simulink model "Torque_Control_22"  (R2023b)
settings: Solver=FixedStepAuto  StartTime=0.0  StopTime=10.0  RelTol=1e-3
libraries: simulink x15, peGeneralControl x6
(part 1 of 6)
settings Model: Creator=cspt  LastModifiedBy=Mátyás
settings SolverCC: AlgebraicLoopSolver=TrustRegion
settings DataIOCC: ReturnWorkspaceOutputs=off
settings DebuggingCC: UnconnectedInputMsg=warning  UnconnectedOutputMsg=warning  UnconnectedLineMsg=warning  ArithmeticOperatorsInVariantConditions=warning
settings ModelReferenceCC: EnableRefExpFcnMdlSchedulingChecks=on
settings SFSimCC: SimUseLocalCustomCode=off  CustomCodeUndefinedFunction=UseInterfaceOnly
settings RTWCC: Description=INTECRIO Real-Time Target  SystemTargetFile=irt.tlc  TemplateMakefile=irt_default_tmf  RTWUseLocalCustomCode=off
settings STFCustomTargetCC: UtilityFuncGeneration=Shared location  GRTInterface=on  SystemTargetFile=irt.tlc
settings GRTTargetCC: UtilityFuncGeneration=Shared location  ParMdlRefBuildCompliant=off  CompOptLevelCompliant=off  ConcurrentExecutionCompliant=off  CombineOutputUpdateFcns=off  MatFileLogging=off  CPPClassGenCompliant=off  GRTInterface=on  UseToolchainInfoCompliant=off  GenerateASAP2=on

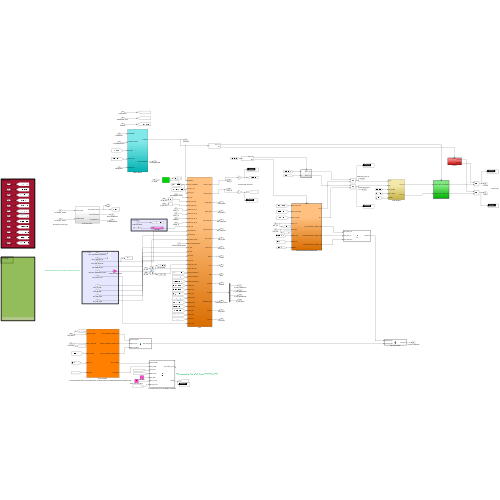
[thumbnail: Simulink's stored preview of the top-level diagram]
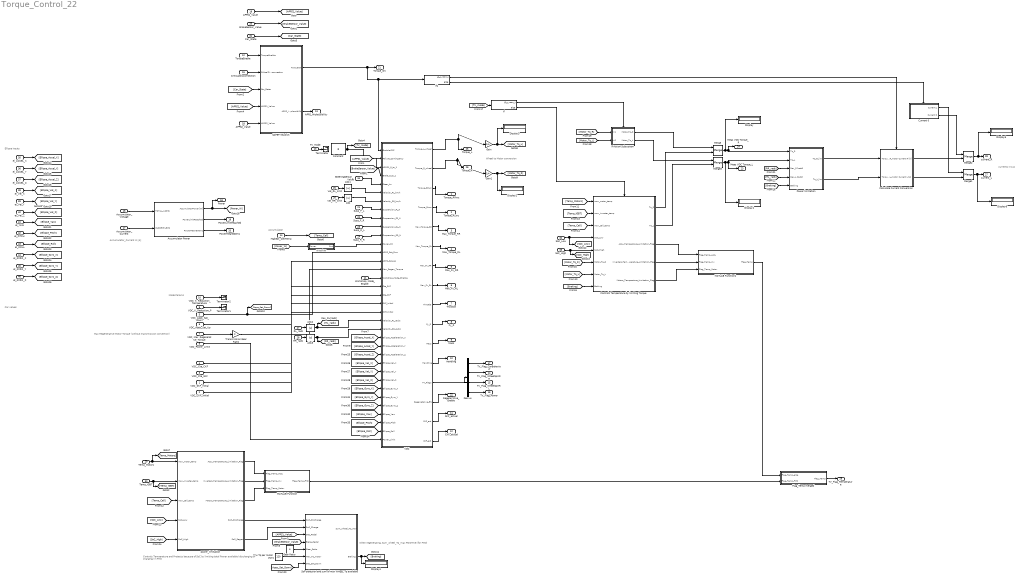
== system Torque_Control_22 ==
  note: Ellipse Inputs
  note: Accumulator_Current in [A]
  note: When regenerating, Sum_wheel_Tq_max POSITIVE (for FM0)
  note: Wheel to Motor conversion
  note: Max Regenerative Motor Torque (without transmission convertion)
  note: Controls Temperature and Protects because of SoC by limiting total Power available (discharging or charging) in FM0
  note: Mode Params
  note: Accumulator
  note: currents in [A]
  note: Car values
  VDC_SKF_Initial : Inport
  VDC_CKF_Initial : Inport  Port=2
  VDC_Cte_SKF : Inport  Port=3
  VDC_Cte_CKF : Inport  Port=4
  VDC_Apps_Sat_Down : Inport  Port=5
  VDC_Apps_Sat_Up : Inport  Port=6
  VDC_Max_Regenerative_Torque : Inport  Port=7
  VDC_Power_Limit : Inport  Port=8
  VDC_K_Reduction_P : Inport  Port=9
  VDC_K_Reduction_Temperature : Inport  Port=10
  Workshop_Mode_Enable : Inport  Port=11
  TorqueEnable : Inport  Port=12
  TV_Mode : Inport  Port=13
  Highest_CellTemp : Inport  Port=14
  CriticalDisconnection : Inport  Port=15
  Accumulator_Voltage : Inport  Port=16
  Accumulator_Current : Inport  Port=17
  APPS2_Value : Inport  Port=18
  APPS1_Value : Inport  Port=19
  BrakeSensor_Value : Inport  Port=20
  Susp_F_L : Inport  Port=21
  Susp_F_R : Inport  Port=22
  Susp_R_L : Inport  Port=23
  Susp_R_R : Inport  Port=24
  Vel_RL_kmh : Inport  Port=25
  Vel_RR_kmh : Inport  Port=26
  RL_rads : Inport  Port=27
  RR_rads : Inport  Port=28
  Temp_Motors : Inport  Port=29
  Temp_IGBT : Inport  Port=30
  Car_State : Inport  Port=31
  SoC_Low : Inport  Port=32
  SoC_High : Inport  Port=33
  SteeringSensor_Value : Inport  Port=34
  el_ACCEL_X : Inport  Port=35
  el_ACCEL_Y : Inport  Port=36
  el_ACCEL_Z : Inport  Port=37
  el_Vel_X : Inport  Port=38
  el_Vel_Y : Inport  Port=39
  el_Vel_Z : Inport  Port=40
  el_YAW : Inport  Port=41
  el_PITCH : Inport  Port=42
  el_ROLL : Inport  Port=43
  el_GYRO_X : Inport  Port=44
  el_GYRO_Y : Inport  Port=45
  el_GYRO_Z : Inport  Port=46
  Abs{,1..3} (4 alike) : Abs  SaturateOnIntegerOverflow=off
  Accumulator Power : Subsystem
  Calculate Current Conversion : Subsystem
  Constant : Constant  Value=3
  Controls Temperature by limiting Torque : Subsystem  TreatAsAtomicUnit=on
  Current 0 : Subsystem  TreatAsAtomicUnit=on
  Demux : Demux
  Display{,1..6} (7 alike) : Display
  Flag_Temp merged : MATLAB Function  TreatAsAtomicUnit=on
  Gain : Gain  Gain=1/4
  Gain1 : Gain  Gain=1/4
  Gear Ratio : Constant  Value=4
  If : If  IfExpression=u1 == 1
  If Action Subsystem : Subsystem  TreatAsAtomicUnit=on
  If1 : If  IfExpression=u1 == 1
  MATLAB Function : MATLAB Function  TreatAsAtomicUnit=on
  MATLAB Function1 : MATLAB Function  TreatAsAtomicUnit=on
  Max Tq per motor [Nm] : Constant  Value=120
  Merge{,1..3} (4 alike) : Merge
  Power limitation : Subsystem
  SAFETY BLOCK : Subsystem
  SoP selection and sum of max WHEEL Tq available : MATLAB Function  TreatAsAtomicUnit=on
  Terminator : Terminator
  Terminator1 : Terminator
  Terminator2 : Terminator
  Transmission Gear Ratio : Gain  Gain=4
  VDC : Subsystem
  W to kW : Subsystem
  power_limitation : Subsystem
  Torque_RRwc : Outport  VectorParamsAs1DForOutWhenUnconnected=off
  Torque_RLwc : Outport  Port=2  VectorParamsAs1DForOutWhenUnconnected=off
  Max_Torque_RR : Outport  Port=3  VectorParamsAs1DForOutWhenUnconnected=off
  Max_Torque_RL : Outport  Port=4  VectorParamsAs1DForOutWhenUnconnected=off
  Max_Fx_RR : Outport  Port=5  VectorParamsAs1DForOutWhenUnconnected=off
  Max_Fx_RL : Outport  Port=6  VectorParamsAs1DForOutWhenUnconnected=off
  Throttle : Outport  Port=7  VectorParamsAs1DForOutWhenUnconnected=off
  Fy_R : Outport  Port=8  VectorParamsAs1DForOutWhenUnconnected=off
  Mass : Outport  Port=9  VectorParamsAs1DForOutWhenUnconnected=off
  Handling : Outport  Port=10  VectorParamsAs1DForOutWhenUnconnected=off
  SKF_actual : Outport  Port=11  VectorParamsAs1DForOutWhenUnconnected=off
  CKF_actual : Outport  Port=12  VectorParamsAs1DForOutWhenUnconnected=off
  APPS_Implausibility : Outport  Port=13  VectorParamsAs1DForOutWhenUnconnected=off
  TV_Flag_WheelSpinRR : Outport  Port=14  VectorParamsAs1DForOutWhenUnconnected=off
  TV_Flag_WheelSpinRL : Outport  Port=15  VectorParamsAs1DForOutWhenUnconnected=off
  TV_Flag_Power : Outport  Port=16  VectorParamsAs1DForOutWhenUnconnected=off
  TV_Flag_CarBehaviour : Outport  Port=17  VectorParamsAs1DForOutWhenUnconnected=off
  Power : Outport  Port=18  VectorParamsAs1DForOutWhenUnconnected=off
  PowerLimitReached : Outport  Port=19  VectorParamsAs1DForOutWhenUnconnected=off
  PowerMean500ms : Outport  Port=20  VectorParamsAs1DForOutWhenUnconnected=off
  Torque_OK : Outport  Port=21  VectorParamsAs1DForOutWhenUnconnected=off
  Regenerative_Enable : Outport  Port=22  VectorParamsAs1DForOutWhenUnconnected=off
  Meas VDC Torque_L : Outport  Port=23  VectorParamsAs1DForOutWhenUnconnected=off
  Meas VDC Torque_R : Outport  Port=24  VectorParamsAs1DForOutWhenUnconnected=off
  Torque_L : Outport  Port=25  VectorParamsAs1DForOutWhenUnconnected=off
  Torque_R : Outport  Port=26  VectorParamsAs1DForOutWhenUnconnected=off
  current_L : Outport  Port=27  VectorParamsAs1DForOutWhenUnconnected=off
  current_R : Outport  Port=28  VectorParamsAs1DForOutWhenUnconnected=off
  TV_Flag_Temperature : Outport  Port=29  VectorParamsAs1DForOutWhenUnconnected=off
  wires:
  Accumulator Power/1(AccumulatorPower [W]) -> [Power_W], Power/1
  Workshop_Mode_Enable/1 -> VDC/16(Workshop_Mode_Enable)
  SAFETY BLOCK/2(APPS_Implausibility) -> APPS_Implausibility/1
  VDC_Cte_SKF/1 -> VDC/18(Cte_CKF)
  VDC_Apps_Sat_Down/1 -> VDC/13(APPS_Sat_Dwn), [Apps_Sat_Down]
  VDC_Cte_CKF/1 -> VDC/17(Cte_SKF)
  VDC_SKF_Initial/1 -> VDC/19(SKF_Initial)
  VDC/3(Torque_RRwc) -> Torque_RRwc/1
  Highest_CellTemp/1 -> [Temp_Cell]
  [Car_State] -> SAFETY BLOCK/3(Car_State)
  Accumulator_Current/1 -> Accumulator Power/2(CURRENT_BMS)
  Accumulator Power/3(PowerMean500ms) -> PowerMean500ms/1
  Demux/1 -> TV_Flag_CarBehaviour/1
  VDC/14(Regenetarive_EN) -> Regenerative_Enable/1
  VDC/10(Fy_R) -> Fy_R/1
  If1/2 -> Current 0/Action
  If1/1 -> Calculate Current Conversion/Action
  VDC_Apps_Sat_Up/1 -> VDC/14(APPS_Sat_Up)
  TorqueEnable/1 -> SAFETY BLOCK/1(TorqueEnable)
  VDC/5(Max_Torque_RR) -> Max_Torque_RR/1
  Accumulator_Voltage/1 -> Accumulator Power/1(TOTAL_V_BMS)
  Accumulator Power/2(PowerLimitReached) -> PowerLimitReached/1
  VDC/7(Max_Fx_RR) -> Max_Fx_RR/1
  VDC/8(Max_Fx_RL) -> Max_Fx_RL/1
  VDC_CKF_Initial/1 -> VDC/20(CKF_Initial)
  Demux/2 -> TV_Flag_WheelSpinRR/1
  VDC/9(Throttle) -> Throttle/1
  Demux/3 -> TV_Flag_WheelSpinRL/1
  [Power_W] -> W to kW/1(Power)
  CriticalDisconnection/1 -> SAFETY BLOCK/2(CriticalDisconnection)
  VDC/11(Mass) -> Mass/1
  VDC/16(CKF_act) -> CKF_actual/1
  VDC/12(Handling) -> Handling/1
  VDC/13(TV_Flags) -> Demux/1
  VDC/6(Max_Torque_RL) -> Max_Torque_RL/1
  VDC/15(SKF_act) -> SKF_actual/1
  VDC/4(Torque_RLwc) -> Torque_RLwc/1
  APPS1_Value/1 -> [APPS1_Value]
  BrakeSensor_Value/1 -> [BrakeSensor_Value]
  Susp_F_L/1 -> VDC/8(Suspension_FL_N)
  Susp_F_R/1 -> VDC/9(Suspension_FR_N)
  Susp_R_L/1 -> VDC/10(Suspension_RL_N)
  Susp_R_R/1 -> VDC/11(Suspension_RR_N)
  APPS2_Value/1 -> SAFETY BLOCK/5(APPS2_Value)
  Car_State/1 -> [Car_State]
  Abs/1 -> VDC/7(Velocity_RR_km/h)
  Abs1/1 -> VDC/6(Velocity_RL_km/h)
  Abs2/1 -> [RL_rads], VDC/21(Velocity_RL_rad/s)
  Merge1/1 -> Display6/1, current_L/1
  Merge2/1 -> Display5/1, current_R/1
  W to kW/1(Out) -> VDC/12(Power_kW)
  VDC/2(Torque_R_wheel) -> Torque_R/1, Gain1/1
  VDC_K_Reduction_P/1 -> Terminator1/1
  VDC_K_Reduction_Temperature/1 -> Terminator2/1
  Demux/4 -> TV_Flag_Power/1
  MATLAB Function/1(Flag_Temp_FM0) -> Flag_Temp merged/2(Flag_Temp_FM0)
  Abs3/1 -> [RR_rads], VDC/22(Velocity_RR_rad/s)
  Current 0/1(Current L) -> Merge1/1
  Calculate Current Conversion/2(Current L [A]) -> Merge1/2
  Transmission Gear Ratio/1 -> VDC/15(Max_Regen_Torque)
  Temp_Motors/1 -> power_limitation/1(max_motor_temp), [Temp_Motors]
  Temp_IGBT/1 -> power_limitation/2(max_inverter_temp), [Temp_IGBT]
  [Temp_Cell] -> power_limitation/3(max_cell_temp)
  [SoC_Low] -> power_limitation/4(SoC_Low)
  [SoC_High] -> power_limitation/5(SoC_High)
  power_limitation/2(Inverters_Temperature_Limitation_Flag) -> MATLAB Function/2(Flag_Temp_Inv)
  power_limitation/1(Accu_Temperature_Limitation_Flag) -> MATLAB Function/1(Flag_Temp_Accu)
  power_limitation/3(Motors_Temperature_Limitation_Flag) -> MATLAB Function/3(Flag_Temp_Motor)
  VDC/1(Torque_L_wheel) -> Gain/1, Torque_L/1
  power_limitation/4(SoP_Discharge) -> SoP selection and sum of max WHEEL Tq available/1(SoP_Discharge)
  power_limitation/5(SoP_Regen) -> SoP selection and sum of max WHEEL Tq available/2(SoP_Charge)
  [APPS1_Value] -> VDC/3(APPS1_0_to_1)
  [BrakeSensor_Value] -> VDC/4(Brake_0_to_1)
  [APPS1_Value] -> SoP selection and sum of max WHEEL Tq available/3(Gas_Pedal)
  [BrakeSensor_Value] -> SoP selection and sum of max WHEEL Tq available/4(Brake_Pedal)
  Gear Ratio/1 -> SoP selection and sum of max WHEEL Tq available/5(Gear_Ratio)
  Max Tq per motor [Nm]/1 -> SoP selection and sum of max WHEEL Tq available/6(Max_Tq_motor)
  [Motor_Tq_R] -> Controls Temperature by limiting Torque/6(Motor_Tq_R)
  [Motor_Tq_L] -> Controls Temperature by limiting Torque/7(Motor_Tq_L)
  MATLAB Function1/1(Flag_Temp) -> Flag_Temp merged/1(Flag_Temp_else)
  [Temp_Motors] -> Controls Temperature by limiting Torque/1(max_motor_temp)
  SoC_High/1 -> [SoC_High], Controls Temperature by limiting Torque/5(SoC_High)
  [Temp_Cell] -> Controls Temperature by limiting Torque/3(max_cell_temp)
  Controls Temperature by limiting Torque/4(Inverters_Temperature_Limitation_Flag) -> MATLAB Function1/2(Flag_Temp_Inv)
  Controls Temperature by limiting Torque/3(Accu_Temperature_Limitation_Flag) -> MATLAB Function1/1(Flag_Temp_Accu)
  [TV_mode] -> If/1
  Gain1/1 -> Display2/1, [Motor_Tq_R]
  Gain/1 -> Display3/1, [Motor_Tq_L]
  Merge3/1 -> Display1/1, Power limitation/2(Tq_L), Meas VDC Torque_L/1
  If/1 -> If Action Subsystem/Action
  [Motor_Tq_R] -> If Action Subsystem/1(In1)
  [Motor_Tq_L] -> If Action Subsystem/2(In2)
  Merge/1 -> Display/1, Power limitation/1(Tq_R), Meas VDC Torque_R/1
  If/2 -> Controls Temperature by limiting Torque/Action
  If Action Subsystem/1(Motor_Tq_R) -> Merge/1
  If Action Subsystem/2(Motor_Tq_L) -> Merge3/1
  Controls Temperature by limiting Torque/1(Tq_R) -> Merge/2
  Controls Temperature by limiting Torque/2(Tq_L) -> Merge3/2
  Flag_Temp merged/1(Flag_Temp) -> TV_Flag_Temperature/1
  Vel_RL_kmh/1 -> Abs1/1
  Vel_RR_kmh/1 -> Abs/1
  RL_rads/1 -> Abs2/1
  RR_rads/1 -> Abs3/1
  VDC_Max_Regenerative_Torque/1 -> Transmission Gear Ratio/1
  SoC_Low/1 -> [SoC_Low], Controls Temperature by limiting Torque/4(SoC_Low)
  [Temp_IGBT] -> Controls Temperature by limiting Torque/2(max_inverter_temp)
  Controls Temperature by limiting Torque/5(Motors_Temperature_Limitation_Flag) -> MATLAB Function1/3(Flag_Temp_Motor)
  [Apps_Sat_Down] -> SoP selection and sum of max WHEEL Tq available/7(Gas_Sat_Down)
  SoP selection and sum of max WHEEL Tq available/2(Braking) -> Display4/1, [Braking]
  [Braking] -> Controls Temperature by limiting Torque/8(Braking)
  Calculate Current Conversion/1(Current R [A]) -> Merge2/2
  Current 0/2(Current R) -> Merge2/1
  SAFETY BLOCK/1(TorqueOK) -> If1/1, VDC/1(EnableVDC), Torque_OK/1
  [RR_rads] -> Power limitation/3(Rev_R [rads])
  [RL_rads] -> Power limitation/4(Rev_L [rads])
  [Braking] -> Power limitation/5(Braking)
  Power limitation/1(Tq_R_lim) -> Calculate Current Conversion/1(Torque_R_motor)
  Power limitation/2(Tq_L_lim) -> Calculate Current Conversion/2(Torque_L_motor)
  TV_Mode/1 -> Terminator/1
  Constant/1 -> [TV_mode], VDC/2(Failure_Contingency)
  SteeringSensor_Value/1 -> VDC/5(Steer_An)
  [APPS1_Value] -> SAFETY BLOCK/4(APPS1_Value)
  el_ACCEL_X/1 -> [Ellipse_Accel_X]
  el_ACCEL_Y/1 -> [Ellipse_Accel_Y]
  el_ACCEL_Z/1 -> [Ellipse_Accel_Z]
  el_Vel_Y/1 -> [Ellipse_Vel_Y]
  el_Vel_Z/1 -> [Ellipse_Vel_Z]
  el_Vel_X/1 -> [Ellipse_Vel_X]
  el_PITCH/1 -> [Ellipse_Pitch]
  el_ROLL/1 -> [Ellipse_Roll]
  el_GYRO_X/1 -> [Ellipse_Gyro_X]
  el_GYRO_Y/1 -> [Ellipse_Gyro_Y]
  el_GYRO_Z/1 -> [Ellipse_Gyro_Z]
  el_YAW/1 -> [Ellipse_Yaw]
  [Ellipse_Accel_X] -> VDC/23(Ellipse_Acceleration_X)
  [Ellipse_Accel_Y] -> VDC/24(Ellipse_Acceleration_Y)
  [Ellipse_Accel_Z] -> VDC/25(Ellipse_Acceleration_Z)
  [Ellipse_Vel_X] -> VDC/26(Ellipse_Vel_X)
  [Ellipse_Vel_Y] -> VDC/27(Ellipse_Vel_Y)
  [Ellipse_Vel_Z] -> VDC/28(Ellipse_Vel_Z)
  [Ellipse_Gyro_X] -> VDC/29(Ellipse_Gyro_X)
  [Ellipse_Gyro_Y] -> VDC/30(Ellipse_Gyro_Y)
  [Ellipse_Gyro_Z] -> VDC/31(Ellipse_Gyro_Z)
  [Ellipse_Yaw] -> VDC/32(Ellipse_Yaw)
  [Ellipse_Pitch] -> VDC/33(Ellipse_Pitch)
  [Ellipse_Roll] -> VDC/34(Ellipse_Roll)
  VDC_Power_Limit/1 -> VDC/35(Power_Limit)

== system Torque_Control_22/Accumulator Power ==
  TOTAL_V_BMS : Inport
  CURRENT_BMS : Inport  Port=2
  PowerLimitDetection : Subsystem  TreatAsAtomicUnit=on
  Product : Product
  AccumulatorPower [W] : Outport  VectorParamsAs1DForOutWhenUnconnected=off
  PowerLimitReached : Outport  Port=2  VectorParamsAs1DForOutWhenUnconnected=off
  PowerMean500ms : Outport  Port=3  VectorParamsAs1DForOutWhenUnconnected=off
  wires:
  Product/1 -> AccumulatorPower [W]/1, PowerLimitDetection/1(Power)
  PowerLimitDetection/1(PowerLimitReached) -> PowerLimitReached/1
  PowerLimitDetection/2(PowerMean500ms) -> PowerMean500ms/1
  TOTAL_V_BMS/1 -> Product/1
  CURRENT_BMS/1 -> Product/2

== system Torque_Control_22/Calculate Current Conversion ==
  Torque_R_motor : Inport
  Torque_L_motor : Inport  Port=2
  Action Port : ActionPort  ActionPortLabel=if { }
  Gain : Gain  Gain=-1
  KT_L_TORKY : Subsystem  TreatAsAtomicUnit=on
  KT_R_EMY : Subsystem  TreatAsAtomicUnit=on
  Current R [A] : Outport  VectorParamsAs1DForOutWhenUnconnected=off
  Current L [A] : Outport  Port=2  VectorParamsAs1DForOutWhenUnconnected=off
  wires:
  Torque_R_motor/1 -> KT_R_EMY/1(Torque)
  Torque_L_motor/1 -> KT_L_TORKY/1(Torque)
  Gain/1 -> Current L [A]/1
  KT_R_EMY/1(Current) -> Current R [A]/1
  KT_L_TORKY/1(Current) -> Gain/1

== system Torque_Control_22/Controls Temperature by limiting Torque ==
  note: Outputs:
      | Flags: 1 means power is being limited by temperature, 0 means not limited
      | SoP_discharge: State of Power for discharging
      | SoP_charge: State of Power for charging
  note: Inputs:
      | max_cell_temp: signal from AMS_Master (Highest_Cell_Temp) [ºC]
      | max_inverter_temp: highest temperature of any of the inverters [ºC]
      | max_motor_temp: highest temperature of any of the motors [ºC]
      | SoC_Low, SoC_High: Lowest & Highest cell state of charge (0-100) [%]
  max_motor_temp : Inport
  max_inverter_temp : Inport  Port=2
  max_cell_temp : Inport  Port=3
  SoC_Low : Inport  Port=4
  SoC_High : Inport  Port=5
  Motor_Tq_R : Inport  Port=6
  Motor_Tq_L : Inport  Port=7
  Braking : Inport  Port=8
  Action Port : ActionPort  ActionPortLabel=else { }
  Max_Tq_per_motor : Constant  Value=120
  Saturation : Saturate  UpperLimit=1  LowerLimit=0
  Saturation1 : Saturate  UpperLimit=1  LowerLimit=0
  SoC_SoP : Subsystem
  Tq_limitation because of Temp : MATLAB Function  TreatAsAtomicUnit=on
  initial_limitation : Constant  Value=0.4
  temperature_SoP : Subsystem
  Tq_R : Outport  VectorParamsAs1DForOutWhenUnconnected=off
  Tq_L : Outport  Port=2  VectorParamsAs1DForOutWhenUnconnected=off
  Accu_Temperature_Limitation_Flag : Outport  Port=3
  Inverters_Temperature_Limitation_Flag : Outport  Port=4
  Motors_Temperature_Limitation_Flag : Outport  Port=5
  wires:
  temperature_SoP/1(SoP) -> SoC_SoP/3(SoP_Temperature)  "temperature_SoP"
  SoC_Low/1 -> SoC_SoP/1(SoC_Low)
  Saturation1/1 -> Tq_limitation because of Temp/2(SoP_Charge)
  SoC_High/1 -> SoC_SoP/2(SoC_High)
  initial_limitation/1 -> temperature_SoP/4(initial_limitation)
  Saturation/1 -> Tq_limitation because of Temp/1(SoP_Discharge)
  temperature_SoP/4(Motors_Temperature_Limitation_Flag) -> Motors_Temperature_Limitation_Flag/1
  temperature_SoP/2(Accu_Temperature_Limitation_Flag) -> Accu_Temperature_Limitation_Flag/1
  SoC_SoP/2(SoP_Regen) -> Saturation1/1  "SoP_Regen"
  max_inverter_temp/1 -> temperature_SoP/2(max_inverter_temp)
  SoC_SoP/1(SoP_Discharge) -> Saturation/1  "SoP_Discharge"
  temperature_SoP/3(Inverters_Temperature_Limitation_Flag) -> Inverters_Temperature_Limitation_Flag/1
  max_cell_temp/1 -> temperature_SoP/3(max_cell_temp), SoC_SoP/4(max_cell_temp)
  max_motor_temp/1 -> temperature_SoP/1(max_motor_temp)
  Braking/1 -> Tq_limitation because of Temp/3(Braking)
  Motor_Tq_R/1 -> Tq_limitation because of Temp/4(Tq_R)
  Motor_Tq_L/1 -> Tq_limitation because of Temp/5(Tq_L)
  Tq_limitation because of Temp/1(Tq_R_limited) -> Tq_R/1
  Tq_limitation because of Temp/2(Tq_L_limited) -> Tq_L/1
  Max_Tq_per_motor/1 -> Tq_limitation because of Temp/6(Max_Tq_per_motor)

== system Torque_Control_22/Current 0 ==
  Action Port : ActionPort  ActionPortLabel=else { }
  Constant : Constant  Value=0
  Current L : Outport  VectorParamsAs1DForOutWhenUnconnected=off
  Current R : Outport  Port=2  VectorParamsAs1DForOutWhenUnconnected=off
  wires:
  Constant/1 -> Current R/1, Current L/1

== system Torque_Control_22/If Action Subsystem ==
  note: Tq already limited (because of Temp and Power) with the SoC
  In1 : Inport
  In2 : Inport  Port=2
  Action Port : ActionPort  ActionPortLabel=if { }
  Motor_Tq_R : Outport  VectorParamsAs1DForOutWhenUnconnected=off
  Motor_Tq_L : Outport  Port=2  VectorParamsAs1DForOutWhenUnconnected=off
  wires:
  In1/1 -> Motor_Tq_R/1
  In2/1 -> Motor_Tq_L/1

== system Torque_Control_22/Power limitation ==
  Tq_R : Inport
  Tq_L : Inport  Port=2
  Rev_R [rads] : Inport  Port=3
  Rev_L [rads] : Inport  Port=4
  Braking : Inport  Port=5
  MATLAB Function : MATLAB Function  TreatAsAtomicUnit=on
  Max_Power_charge [kW] : Constant  Value=60
  Max_Power_discharge [kW] : Constant  Value=80
  Tq_R_lim : Outport  VectorParamsAs1DForOutWhenUnconnected=off
  Tq_L_lim : Outport  Port=2  VectorParamsAs1DForOutWhenUnconnected=off
  wires:
  Tq_R/1 -> MATLAB Function/1(Tq_R)
  Tq_L/1 -> MATLAB Function/2(Tq_L)
  Rev_R [rads]/1 -> MATLAB Function/3(Rev_R)
  Rev_L [rads]/1 -> MATLAB Function/4(Rev_L)
  Braking/1 -> MATLAB Function/5(Braking)
  Max_Power_discharge [kW]/1 -> MATLAB Function/6(Max_Power_Discharge)
  Max_Power_charge [kW]/1 -> MATLAB Function/7(Max_Power_Charge)
  MATLAB Function/1(Tq_R_lim) -> Tq_R_lim/1
  MATLAB Function/2(Tq_L_lim) -> Tq_L_lim/1

== system Torque_Control_22/SAFETY BLOCK ==
  note: Añandir último elemento cadena del BMS
  note: CriticalDisconnection -> 1
      | OK -> 0
  TorqueEnable : Inport
  CriticalDisconnection : Inport  Port=2
  Car_State : Inport  Port=3
  APPS1_Value : Inport  Port=4
  APPS2_Value : Inport  Port=5
  APPS_IMPLAUSIBILITY : Subsystem
  Compare To Constant : simulink/Logic and Bit Operations/Compare To Constant  relop===  const=15  OutDataTypeStr=boolean
  Logical Operator : Logic  Inputs=5  OutDataTypeStr=boolean
  Logical Operator1 : Logic  Operator=NOT  IconShape=distinctive  AllPortsSameDT=off  OutDataTypeStr=boolean
  NOT : Logic  Operator=NOT  IconShape=distinctive  AllPortsSameDT=off  OutDataTypeStr=boolean
  TorqueOK : Outport  VectorParamsAs1DForOutWhenUnconnected=off
  APPS_Implausibility : Outport  Port=2  VectorParamsAs1DForOutWhenUnconnected=off
  wires:
  Logical Operator/1 -> TorqueOK/1
  Car_State/1 -> Compare To Constant/1
  NOT/1 -> Logical Operator/3
  CriticalDisconnection/1 -> NOT/1
  TorqueEnable/1 -> Logical Operator/2
  APPS2_Value/1 -> APPS_IMPLAUSIBILITY/2(APPS2)
  APPS1_Value/1 -> APPS_IMPLAUSIBILITY/1(APPS1)
  Logical Operator1/1 -> APPS_Implausibility/1
  Compare To Constant/1 -> Logical Operator/4
  APPS_IMPLAUSIBILITY/1(OK) -> Logical Operator/5, Logical Operator1/1

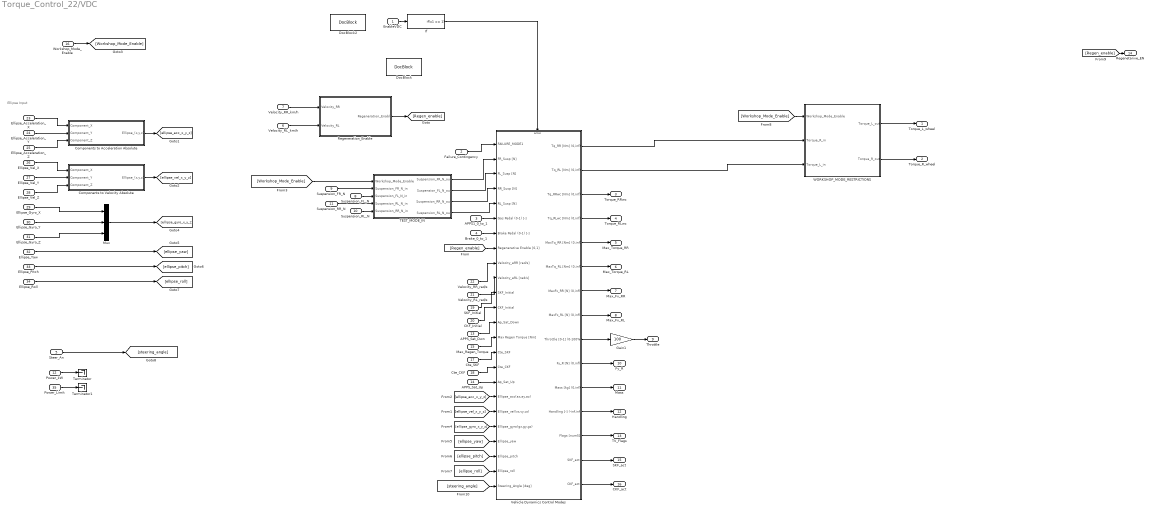
== system Torque_Control_22/VDC ==
  note: Ellipse Input
  EnableVDC : Inport
  Failure_Contingency : Inport  Port=2
  APPS1_0_to_1 : Inport  Port=3
  Brake_0_to_1 : Inport  Port=4
  Steer_An : Inport  Port=5
  Velocity_RL_km/h : Inport  Port=6
  Velocity_RR_km/h : Inport  Port=7
  Suspension_FL_N : Inport  Port=8
  Suspension_FR_N : Inport  Port=9
  Suspension_RL_N : Inport  Port=10
  Suspension_RR_N : Inport  Port=11
  Power_kW : Inport  Port=12
  APPS_Sat_Dwn : Inport  Port=13
  APPS_Sat_Up : Inport  Port=14
  Max_Regen_Torque : Inport  Port=15
  Workshop_Mode_Enable : Inport  Port=16
  Cte_SKF : Inport  Port=17
  Cte_CKF : Inport  Port=18
  SKF_Initial : Inport  Port=19
  CKF_Initial : Inport  Port=20
  Velocity_RL_rad/s : Inport  Port=21
  Velocity_RR_rad/s : Inport  Port=22
  Ellipse_Acceleration_X : Inport  Port=23
  Ellipse_Acceleration_Y : Inport  Port=24
  Ellipse_Acceleration_Z : Inport  Port=25
  Ellipse_Vel_X : Inport  Port=26
  Ellipse_Vel_Y : Inport  Port=27
  Ellipse_Vel_Z : Inport  Port=28
  Ellipse_Gyro_X : Inport  Port=29
  Ellipse_Gyro_Y : Inport  Port=30
  Ellipse_Gyro_Z : Inport  Port=31
  Ellipse_Yaw : Inport  Port=32
  Ellipse_Pitch : Inport  Port=33
  Ellipse_Roll : Inport  Port=34
  Power_Limit : Inport  Port=35
  Components to Acceleration Absolute : Subsystem
  Components to Velocity Absolute : Subsystem
  DocBlock : simulink/Model-Wide Utilities/DocBlock  DocumentType=Text
      content=|
      | This port activates the different modes that the VDC must be in according
      | to the signals that the Main ECU has available.
      |
      | Port Must be 1 to activate VDC 2018 Complete (Green)
      | Requirement: All sensors are connected (Ellipse, Steering, SuspensionRear
      | [SuspensionFront only needed to calculate Mass]).
      |
      | Port Must be 2 to activate VDC without Longitudinal (Yellow)
      | Requirement: No steering sensor data
      |
      | Port Must be 3 to activate Steering TV 2017 without TC (Orange)
      | Requirement: (No Ellipse) or (No SuspensionRear Data)
      |
      | Port Must be 4 to activate Rigid Axle (Red)
      | Requirement: (No Steering Sensor) and (No Ellipse or No SuspensionRear)
  DocBlock2 : simulink/Model-Wide Utilities/DocBlock  DocumentType=Text
      content=|
      | Enable Vehicle Dynamics Control.
      |
      | This port must be 1 if the calculations for VDC must be made
  Gain1 : Gain  Gain=100
  If : If  IfExpression=u1 == 1  ShowElse=off
  Mux : Mux  Inputs=3
  Regeneration_Enable : Subsystem  TreatAsAtomicUnit=on
  TEST_MODE_IN : Subsystem  TreatAsAtomicUnit=on
  Terminator : Terminator
  Terminator1 : Terminator
  Vehicle Dynamics Control Modes : Subsystem
  WORKSHOP_MODE_RESTRICTIONS : Subsystem  TreatAsAtomicUnit=on
  Torque_L_wheel : Outport  VectorParamsAs1DForOutWhenUnconnected=off
  Torque_R_wheel : Outport  Port=2  VectorParamsAs1DForOutWhenUnconnected=off
  Torque_RRwc : Outport  Port=3  VectorParamsAs1DForOutWhenUnconnected=off
  Torque_RLwc : Outport  Port=4  VectorParamsAs1DForOutWhenUnconnected=off
  Max_Torque_RR : Outport  Port=5  VectorParamsAs1DForOutWhenUnconnected=off
  Max_Torque_RL : Outport  Port=6  VectorParamsAs1DForOutWhenUnconnected=off
  Max_Fx_RR : Outport  Port=7  VectorParamsAs1DForOutWhenUnconnected=off
  Max_Fx_RL : Outport  Port=8  VectorParamsAs1DForOutWhenUnconnected=off
  Throttle : Outport  Port=9  VectorParamsAs1DForOutWhenUnconnected=off
  Fy_R : Outport  Port=10  VectorParamsAs1DForOutWhenUnconnected=off
  Mass : Outport  Port=11  VectorParamsAs1DForOutWhenUnconnected=off
  Handling : Outport  Port=12  VectorParamsAs1DForOutWhenUnconnected=off
  TV_Flags : Outport  Port=13  VectorParamsAs1DForOutWhenUnconnected=off
  Regenetarive_EN : Outport  Port=14  VectorParamsAs1DForOutWhenUnconnected=off
  SKF_act : Outport  Port=15  VectorParamsAs1DForOutWhenUnconnected=off
  CKF_act : Outport  Port=16  VectorParamsAs1DForOutWhenUnconnected=off
  wires:
  Velocity_RR_km/h/1 -> Regeneration_Enable/1(Velocity_RR)
  Gain1/1 -> Throttle/1
  Vehicle Dynamics Control Modes/7(MaxFx_RR [N] (0,inf)) -> Max_Fx_RR/1
  Vehicle Dynamics Control Modes/6(MaxTq_RL [Nm] (0,inf)) -> Max_Torque_RL/1
  Vehicle Dynamics Control Modes/8(MaxFx_RL [N] (0,inf)) -> Max_Fx_RL/1
  Power_kW/1 -> Terminator/1
  Vehicle Dynamics Control Modes/1(Tq_RR [Nm] (0,inf)) -> WORKSHOP_MODE_RESTRICTIONS/2(Torque_R_in)
  APPS_Sat_Up/1 -> Vehicle Dynamics Control Modes/17(Ap_Sat_Up)
  WORKSHOP_MODE_RESTRICTIONS/1(Torque_L_out) -> Torque_L_wheel/1
  Vehicle Dynamics Control Modes/3(Tq_RRwc [Nm] (0,inf)) -> Torque_RRwc/1
  Suspension_FL_N/1 -> TEST_MODE_IN/3(Suspension_FL_N_in)
  Suspension_FR_N/1 -> TEST_MODE_IN/2(Suspension_FR_N_in)
  TEST_MODE_IN/1(Suspension_FR_N_out) -> Vehicle Dynamics Control Modes/2(FR_Susp [N])
  Velocity_RR_rad/s/1 -> Vehicle Dynamics Control Modes/9(Velocity_eRR [rad/s])
  Vehicle Dynamics Control Modes/14(SKF_act) -> SKF_act/1
  APPS1_0_to_1/1 -> Vehicle Dynamics Control Modes/6(Gas Pedal (0-1) [-])
  Vehicle Dynamics Control Modes/4(Tq_RLwc [Nm] (0,inf)) -> Torque_RLwc/1
  Vehicle Dynamics Control Modes/5(MaxTq_RR [Nm] (0,inf)) -> Max_Torque_RR/1
  Brake_0_to_1/1 -> Vehicle Dynamics Control Modes/7(Brake Pedal (0-1) [-])
  Velocity_RL_km/h/1 -> Regeneration_Enable/2(Velocity_RL)
  Vehicle Dynamics Control Modes/11(Mass [kg] (0,inf)) -> Mass/1
  Vehicle Dynamics Control Modes/9(Throttle [0-1] (0-100%)) -> Gain1/1
  Vehicle Dynamics Control Modes/2(Tq_RL [Nm] (0,inf)) -> WORKSHOP_MODE_RESTRICTIONS/3(Torque_L_in)
  EnableVDC/1 -> If/1
  Suspension_RL_N/1 -> TEST_MODE_IN/5(Suspension_RR_N_in)
  Vehicle Dynamics Control Modes/10(Fy_R [N] (0,inf)) -> Fy_R/1
  Vehicle Dynamics Control Modes/13(Flags [num5]) -> TV_Flags/1
  [Workshop_Mode_Enable] -> TEST_MODE_IN/1(Workshop_Mode_Enable)
  Suspension_RR_N/1 -> TEST_MODE_IN/4(Suspension_RL_N_in)
  Vehicle Dynamics Control Modes/12(Handling [-] (-inf,inf)) -> Handling/1
  Workshop_Mode_Enable/1 -> [Workshop_Mode_Enable]
  Vehicle Dynamics Control Modes/15(CKF_act) -> CKF_act/1
  If/1 -> Vehicle Dynamics Control Modes/Action
  TEST_MODE_IN/2(Suspension_FL_N_out) -> Vehicle Dynamics Control Modes/3(FL_Susp [N])
  TEST_MODE_IN/3(Suspension_RR_N_out) -> Vehicle Dynamics Control Modes/4(RR_Susp [N])
  TEST_MODE_IN/4(Suspension_RL_N_out) -> Vehicle Dynamics Control Modes/5(RL_Susp [N])
  Velocity_RL_rad/s/1 -> Vehicle Dynamics Control Modes/10(Velocity_eRL [rad/s])
  SKF_Initial/1 -> Vehicle Dynamics Control Modes/11(SKF_Initial)
  CKF_Initial/1 -> Vehicle Dynamics Control Modes/12(CKF_Initial)
  APPS_Sat_Dwn/1 -> Vehicle Dynamics Control Modes/13(Ap_Sat_Down)
  Max_Regen_Torque/1 -> Vehicle Dynamics Control Modes/14(Max Regen Torque [Nm])
  Cte_SKF/1 -> Vehicle Dynamics Control Modes/15(Cte_SKF)
  Cte_CKF/1 -> Vehicle Dynamics Control Modes/16(Cte_CKF)
  Failure_Contingency/1 -> Vehicle Dynamics Control Modes/1(FAILURE_MODE1)
  Regeneration_Enable/1(Regeneration_Enable) -> [Regen_enable]
  [Regen_enable] -> Vehicle Dynamics Control Modes/8(Regenerative Enable [0,1])
  WORKSHOP_MODE_RESTRICTIONS/2(Torque_R_out) -> Torque_R_wheel/1
  Components to Acceleration Absolute/1(Ellipse_(x,y,z)) -> [ellipse_acc_x_y_z]
  Ellipse_Acceleration_X/1 -> Components to Acceleration Absolute/1(Component_X)
  Ellipse_Acceleration_Y/1 -> Components to Acceleration Absolute/2(Component_Y)
  Ellipse_Acceleration_Z/1 -> Components to Acceleration Absolute/3(Component_Z)
  Components to Velocity Absolute/1(Ellipse_(x,y,z)) -> [ellipse_vel_x_y_z]
  Ellipse_Vel_X/1 -> Components to Velocity Absolute/1(Component_X)
  Ellipse_Vel_Z/1 -> Components to Velocity Absolute/3(Component_Z)
  Ellipse_Vel_Y/1 -> Components to Velocity Absolute/2(Component_Y)
  Ellipse_Gyro_X/1 -> Mux/1
  Ellipse_Gyro_Y/1 -> Mux/2
  Ellipse_Gyro_Z/1 -> Mux/3
  Mux/1 -> [ellipse_gyro_x_y_z]
  Ellipse_Yaw/1 -> [ellipse_yaw]
  Ellipse_Pitch/1 -> [ellipse_pitch]
  Ellipse_Roll/1 -> [ellipse_roll]
  [ellipse_vel_x_y_z] -> Vehicle Dynamics Control Modes/19(Ellipse_vel(vx,vy,vz))
  [ellipse_acc_x_y_z] -> Vehicle Dynamics Control Modes/18(Ellipse_acc(ax,ay,az))
  [ellipse_gyro_x_y_z] -> Vehicle Dynamics Control Modes/20(Ellipse_gyro(gx,gy,gz))
  [ellipse_yaw] -> Vehicle Dynamics Control Modes/21(Ellipse_yaw)
  [ellipse_pitch] -> Vehicle Dynamics Control Modes/22(Ellipse_pitch)
  [ellipse_roll] -> Vehicle Dynamics Control Modes/23(Ellipse_roll)
  [Workshop_Mode_Enable] -> WORKSHOP_MODE_RESTRICTIONS/1(Workshop_Mode_Enable)
  [Regen_enable] -> Regenetarive_EN/1
  Steer_An/1 -> [steering_angle]
  [steering_angle] -> Vehicle Dynamics Control Modes/24(Steering_Angle [deg])
  Power_Limit/1 -> Terminator1/1

== system Torque_Control_22/W to kW ==
  Power : Inport
  0-100 to 0-2 : Constant  Value=1000
  Divide5 : Product  Inputs=*/
  Out : Outport  VectorParamsAs1DForOutWhenUnconnected=off
  wires:
  Power/1 -> Divide5/1
  0-100 to 0-2/1 -> Divide5/2
  Divide5/1 -> Out/1

== system Torque_Control_22/power_limitation ==
  note: Inputs:
      | max_cell_temp: signal from AMS_Master (Highest_Cell_Temp) [ºC]
      | max_inverter_temp: highest temperature of any of the inverters [ºC]
      | max_motor_temp: highest temperature of any of the motors [ºC]
      | SoC_Low, SoC_High: Lowest & Highest cell state of charge (0-100) [%]
  note: Outputs:
      | Flags: 1 means power is being limited by temperature, 0 means not limited
      | SoP_discharge: State of Power for discharging
      | SoP_charge: State of Power for charging
  max_motor_temp : Inport
  max_inverter_temp : Inport  Port=2
  max_cell_temp : Inport  Port=3
  SoC_Low : Inport  Port=4
  SoC_High : Inport  Port=5
  Saturation : Saturate  UpperLimit=1  LowerLimit=0
  Saturation1 : Saturate  UpperLimit=1  LowerLimit=0
  SoC_SoP : Subsystem
  initial_limitation : Constant  Value=0.4
  temperature_SoP : Subsystem
  Accu_Temperature_Limitation_Flag : Outport
  Inverters_Temperature_Limitation_Flag : Outport  Port=2
  Motors_Temperature_Limitation_Flag : Outport  Port=3
  SoP_Discharge : Outport  Port=4
  SoP_Regen : Outport  Port=5
  wires:
  SoC_SoP/1(SoP_Discharge) -> Saturation/1  "SoP_Discharge"
  SoC_SoP/2(SoP_Regen) -> Saturation1/1  "SoP_Regen"
  max_motor_temp/1 -> temperature_SoP/1(max_motor_temp)
  max_inverter_temp/1 -> temperature_SoP/2(max_inverter_temp)
  max_cell_temp/1 -> temperature_SoP/3(max_cell_temp), SoC_SoP/4(max_cell_temp)
  initial_limitation/1 -> temperature_SoP/4(initial_limitation)
  temperature_SoP/1(SoP) -> SoC_SoP/3(SoP_Temperature)  "temperature_SoP"
  temperature_SoP/4(Motors_Temperature_Limitation_Flag) -> Motors_Temperature_Limitation_Flag/1
  temperature_SoP/3(Inverters_Temperature_Limitation_Flag) -> Inverters_Temperature_Limitation_Flag/1
  temperature_SoP/2(Accu_Temperature_Limitation_Flag) -> Accu_Temperature_Limitation_Flag/1
  SoC_High/1 -> SoC_SoP/2(SoC_High)
  SoC_Low/1 -> SoC_SoP/1(SoC_Low)
  Saturation/1 -> SoP_Discharge/1
  Saturation1/1 -> SoP_Regen/1

== system Torque_Control_22/Accumulator Power/PowerLimitDetection ==
  note: mean:500ms
      | time:25ms
      | moving window: 500/25=20
  Power : Inport
  Data Store Memory10 : DataStoreMemory  ReadBeforeWriteMsg=warning  WriteAfterWriteMsg=warning  WriteAfterReadMsg=warning  ShowAdditionalParam=off
  Data Store Read30 : DataStoreRead  IndexOptions=Index vector (dialog)  Indices=1  OutputSizes=1
  Data Store Write20 : DataStoreWrite  IndexOptions=Index vector (dialog)  Indices=1  OutputSizes=1
  If : If  IfExpression=u1 >= 80000
  LimitReached : Subsystem  TreatAsAtomicUnit=on
  Merge1 : Merge
  OK_OrLatch : Subsystem  TreatAsAtomicUnit=on
  PowerLimitReached : Outport  VectorParamsAs1DForOutWhenUnconnected=off
  PowerMean500ms : Outport  Port=2  VectorParamsAs1DForOutWhenUnconnected=off
  wires:
  Power/1 -> If/1, PowerMean500ms/1
  If/1 -> LimitReached/Action
  If/2 -> OK_OrLatch/Action
  LimitReached/1("Out ") -> Merge1/1
  OK_OrLatch/1(Out 1) -> Merge1/2
  Merge1/1 -> Data Store Write20/1, PowerLimitReached/1
  Data Store Read30/1 -> OK_OrLatch/1(IN)

== system Torque_Control_22/Calculate Current Conversion/KT_L_TORKY ==
  Torque : Inport
  A/Nm : Gain  Gain=0.2
  Current : Outport  VectorParamsAs1DForOutWhenUnconnected=off
  wires:
  A/Nm/1 -> Current/1
  Torque/1 -> A/Nm/1

== system Torque_Control_22/Calculate Current Conversion/KT_R_EMY ==
  Torque : Inport
  A/Nm : Gain  Gain=0.2
  Current : Outport  VectorParamsAs1DForOutWhenUnconnected=off
  wires:
  Torque/1 -> A/Nm/1
  A/Nm/1 -> Current/1

== system Torque_Control_22/Controls Temperature by limiting Torque/SoC_SoP ==
  note: El lookup se puede obtener ensayando una celda en una descarga y en una carga con pérdidas de calor constantes. La corriente normalizada será el lookup.
  note: Si está descargada, no descargues más
  note: Si está cargada, no
      | cargues más
  SoC_Low : Inport
  SoC_High : Inport  Port=2
  SoP_Temperature : Inport  Port=3
  max_cell_temp : Inport  Port=4
  Gain5 : Gain  Gain=1/100
  Gain6 : Gain  Gain=1/100
  Lookup_SoC_SoP_chg : Lookup_n-D  NumberOfTableDimensions=1  BreakpointsForDimension1=[0.02 0.1 0.2 0.3 0.5 0.8 0.95 1]  Table=[0.95 1 1 1 1 0.9 0.75 0.02]  InternalRulePriority=Speed  RndMeth=Simplest
  Lookup_SoC_SoP_dischg : Lookup_n-D  NumberOfTableDimensions=1  BreakpointsForDimension1=[0.02 0.1 0.2 0.3 0.5 0.8 0.9 1]  Table=[0.4 0.6 0.8 0.95 1 1 0.98 0.95]  InternalRulePriority=Speed  RndMeth=Simplest
  Lookup_Temp_SoP_chg : Lookup_n-D  NumberOfTableDimensions=1  BreakpointsForDimension1=[45 48 49 50 51]  Table=[1 0.75 0.5 0 0]  InternalRulePriority=Speed  RndMeth=Simplest
  Product : Product
  Product4 : Product
  Product5 : Product
  SoP_Discharge : Outport
  SoP_Regen : Outport  Port=2
  wires:
  Lookup_SoC_SoP_dischg/1 -> Product4/1
  Product/1 -> Product5/2
  SoP_Temperature/1 -> Product4/2, Product5/1
  SoC_Low/1 -> Gain6/1
  Gain6/1 -> Lookup_SoC_SoP_dischg/1
  SoC_High/1 -> Gain5/1
  Gain5/1 -> Lookup_SoC_SoP_chg/1
  Product5/1 -> SoP_Regen/1
  Product4/1 -> SoP_Discharge/1
  Lookup_SoC_SoP_chg/1 -> Product/1
  max_cell_temp/1 -> Lookup_Temp_SoP_chg/1
  Lookup_Temp_SoP_chg/1 -> Product/2

== system Torque_Control_22/Controls Temperature by limiting Torque/temperature_SoP ==
  max_motor_temp : Inport
  max_inverter_temp : Inport  Port=2
  max_cell_temp : Inport  Port=3
  initial_limitation : Inport  Port=4
  Flag_Accu : simulink/Logic and Bit Operations/Compare To Constant  relop=<  const=1  OutDataTypeStr=boolean  ZeroCross=off
  Flag_Inv : simulink/Logic and Bit Operations/Compare To Constant  relop=<  const=1  OutDataTypeStr=boolean  ZeroCross=off
  Flag_Mot : simulink/Logic and Bit Operations/Compare To Constant  relop=<  const=1  OutDataTypeStr=boolean  ZeroCross=off
  Min : MinMax  Inputs=3
  temperature_rise_limitator_Accu : Subsystem
  temperature_rise_limitator_Inverters : Subsystem
  temperature_rise_limitator_Motors : Subsystem
  SoP : Outport
  Accu_Temperature_Limitation_Flag : Outport  Port=2
  Inverters_Temperature_Limitation_Flag : Outport  Port=3
  Motors_Temperature_Limitation_Flag : Outport  Port=4
  wires:
  temperature_rise_limitator_Inverters/1(SoP) -> Flag_Inv/1, Min/2
  initial_limitation/1 -> temperature_rise_limitator_Accu/2(initial_limitation), temperature_rise_limitator_Motors/2(initial_limitation), temperature_rise_limitator_Inverters/2(initial_limitation)
  Flag_Accu/1 -> Accu_Temperature_Limitation_Flag/1
  temperature_rise_limitator_Motors/1(SoP) -> Flag_Mot/1, Min/3
  max_cell_temp/1 -> temperature_rise_limitator_Accu/1(max_cell_temp)
  temperature_rise_limitator_Accu/1(SoP) -> Flag_Accu/1, Min/1
  Min/1 -> SoP/1
  Flag_Inv/1 -> Inverters_Temperature_Limitation_Flag/1
  Flag_Mot/1 -> Motors_Temperature_Limitation_Flag/1
  max_inverter_temp/1 -> temperature_rise_limitator_Inverters/1(max_inverter_temp)
  max_motor_temp/1 -> temperature_rise_limitator_Motors/1(max_motor_temp)

== system Torque_Control_22/SAFETY BLOCK/APPS_IMPLAUSIBILITY ==
  APPS1 : Inport
  APPS2 : Inport  Port=2
  Ab : Abs  SaturateOnIntegerOverflow=off
  If : If  IfExpression=u1 > 0.1
  Imp : Subsystem  TreatAsAtomicUnit=on
  Merge : Merge
  Not Imp : Subsystem  TreatAsAtomicUnit=on
  Sum : Sum  Inputs=|+-
  OK : Outport  VectorParamsAs1DForOutWhenUnconnected=off
  wires:
  APPS1/1 -> Sum/1
  APPS2/1 -> Sum/2
  Sum/1 -> Ab/1
  Ab/1 -> If/1
  Imp/1(Out1) -> Merge/1  "Bool 0"
  Not Imp/1(Out1) -> Merge/2  "Bool 1"
  Merge/1 -> OK/1
  If/2 -> Not Imp/Action
  If/1 -> Imp/Action

== system Torque_Control_22/VDC/Components to Acceleration Absolute ==
  Component_X : Inport
  Component_Y : Inport  Port=2
  Component_Z : Inport  Port=3
  Abs : Abs  SaturateOnIntegerOverflow=off
  Mux : Mux  Inputs=3
  Ellipse_(x,y,z) : Outport
  wires:
  Abs/1 -> Ellipse_(x,y,z)/1
  Component_Z/1 -> Mux/3
  Component_Y/1 -> Mux/2
  Mux/1 -> Abs/1
  Component_X/1 -> Mux/1

== system Torque_Control_22/VDC/Components to Velocity Absolute ==
  Component_X : Inport
  Component_Y : Inport  Port=2
  Component_Z : Inport  Port=3
  Abs : Abs  SaturateOnIntegerOverflow=off
  Mux : Mux  Inputs=3
  Ellipse_(x,y,z) : Outport
  wires:
  Abs/1 -> Ellipse_(x,y,z)/1
  Component_Z/1 -> Mux/3
  Component_Y/1 -> Mux/2
  Mux/1 -> Abs/1
  Component_X/1 -> Mux/1

== system Torque_Control_22/VDC/Regeneration_Enable ==
  note: Regen is Enable if velocity is higher than 2 km/h, to avoid backwards velocity due to Regen Tq (negative)
  Velocity_RR : Inport
  Velocity_RL : Inport  Port=2
  Enabled : Constant
  "Enabled " : Subsystem  TreatAsAtomicUnit=on
  If : If  NumInputs=2  IfExpression=(u1>2)&(u2>2)
  Merge1 : Merge
  NotEnabled : Subsystem  TreatAsAtomicUnit=on
  "Zero " : Constant  Value=0
  Regeneration_Enable : Outport  VectorParamsAs1DForOutWhenUnconnected=off
  wires:
  Merge1/1 -> Regeneration_Enable/1
  Velocity_RR/1 -> If/1
  Velocity_RL/1 -> If/2
  If/1 -> "Enabled "/Action
  If/2 -> NotEnabled/Action
  "Zero "/1 -> NotEnabled/1(In1)
  NotEnabled/1(Out1) -> Merge1/2
  "Enabled "/1(Out1) -> Merge1/1
  Enabled/1 -> "Enabled "/1(In1)

== system Torque_Control_22/VDC/TEST_MODE_IN ==
  Workshop_Mode_Enable : Inport
  Suspension_FR_N_in : Inport  Port=2
  Suspension_FL_N_in : Inport  Port=3
  Suspension_RL_N_in : Inport  Port=4
  Suspension_RR_N_in : Inport  Port=5
  BYPASS : Subsystem  TreatAsAtomicUnit=on
  If : If  IfExpression=u1 == 1
  Merge{,1..3} (4 alike) : Merge
  TEST_CONSTANTS : Subsystem  TreatAsAtomicUnit=on
  Suspension_FR_N_out : Outport  VectorParamsAs1DForOutWhenUnconnected=off
  Suspension_FL_N_out : Outport  Port=2  VectorParamsAs1DForOutWhenUnconnected=off
  Suspension_RR_N_out : Outport  Port=3  VectorParamsAs1DForOutWhenUnconnected=off
  Suspension_RL_N_out : Outport  Port=4  VectorParamsAs1DForOutWhenUnconnected=off
  wires:
  Suspension_FR_N_in/1 -> BYPASS/1(In1)
  Suspension_FL_N_in/1 -> BYPASS/2(In2)
  Suspension_RR_N_in/1 -> BYPASS/3(In3)
  Suspension_RL_N_in/1 -> BYPASS/4(In4)
  Merge/1 -> Suspension_FR_N_out/1
  Merge1/1 -> Suspension_FL_N_out/1
  Merge2/1 -> Suspension_RR_N_out/1
  Merge3/1 -> Suspension_RL_N_out/1
  BYPASS/1(Out1) -> Merge/1
  BYPASS/2(Out2) -> Merge1/1
  BYPASS/3(Out3) -> Merge2/1
  BYPASS/4(Out4) -> Merge3/1
  Workshop_Mode_Enable/1 -> If/1
  If/2 -> BYPASS/Action
  If/1 -> TEST_CONSTANTS/Action
  TEST_CONSTANTS/4(Out4) -> Merge3/2
  TEST_CONSTANTS/3(Out3) -> Merge2/2
  TEST_CONSTANTS/2(Out2) -> Merge1/2
  TEST_CONSTANTS/1(Out1) -> Merge/2

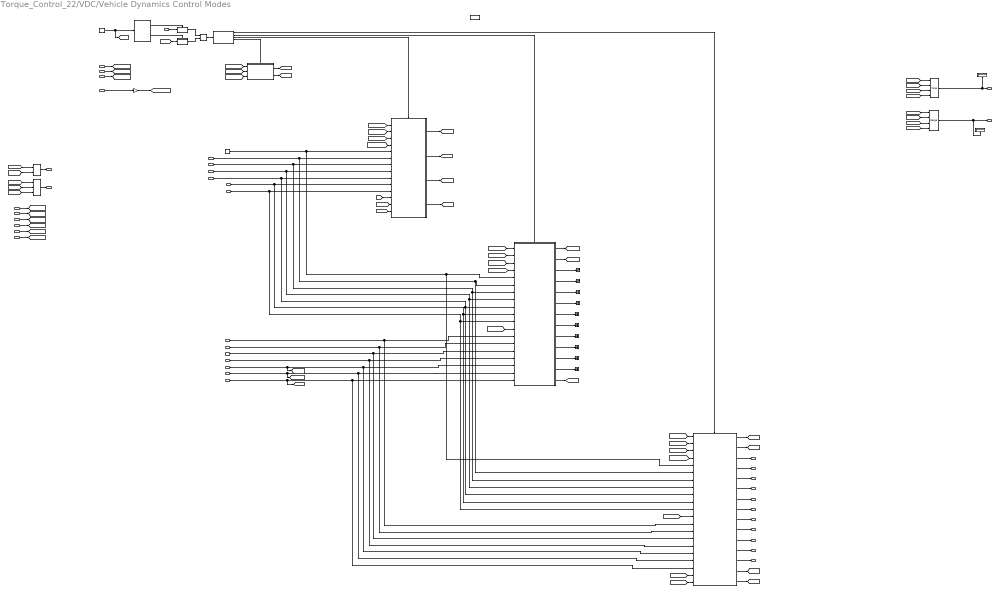
== system Torque_Control_22/VDC/Vehicle Dynamics Control Modes ==
  note: Handling now is negligible is always 0
  note: Ellipse Inputs
  note: Failure Mode Selection: 5 -> Automatic Failure Mode Selection according to sensors available
      | 4 -> Rigid Axle (red)
      | 3 -> Steering TV with TC (orange)
      | 2 -> VDC without longitudinal (yellow)
      | 1 -> VDC complete (green)
      | 0 -> TV with TC 2023
  FAILURE_MODE1 : Inport
  FR_Susp [N] : Inport  Port=2
  FL_Susp [N] : Inport  Port=3
  RR_Susp [N] : Inport  Port=4
  RL_Susp [N] : Inport  Port=5
  Gas Pedal (0-1) [-] : Inport  Port=6
  Brake Pedal (0-1) [-] : Inport  Port=7
  Regenerative Enable [0,1] : Inport  Port=8
  Velocity_eRR [rad/s] : Inport  Port=9
  Velocity_eRL [rad/s] : Inport  Port=10
  SKF_Initial : Inport  Port=11
  CKF_Initial : Inport  Port=12
  Ap_Sat_Down : Inport  Port=13
  Max Regen Torque [Nm] : Inport  Port=14
  Cte_SKF : Inport  Port=15
  Cte_CKF : Inport  Port=16
  Ap_Sat_Up : Inport  Port=17
  Ellipse_acc(ax,ay,az) : Inport  Port=18
  Ellipse_vel(vx,vy,vz) : Inport  Port=19
  Ellipse_gyro(gx,gy,gz) : Inport  Port=20
  Ellipse_yaw : Inport  Port=21
  Ellipse_pitch : Inport  Port=22
  Ellipse_roll : Inport  Port=23
  Steering_Angle [deg] : Inport  Port=24
  Action Port : ActionPort  ActionPortLabel=if { }
  Automatic Failure Mode : Subsystem  TreatAsAtomicUnit=on
  Constant : Constant  Value=5
  Display : Display
  Display1 : Display
  FAILURE MODE : If  IfExpression=u1 == 1  ElseIfExpressions=u1 == 2, u1 == 3, u1 == 4, u1 == 0  ShowElse=off
  Gain : Gain  Gain=-1
  If : If  IfExpression=u1 == 5
  Manual Failure Mode Selection : Subsystem  TreatAsAtomicUnit=on
  Merge : Merge
  Merge Tq_RL : Merge  Inputs=4
  Merge Tq_RR : Merge  Inputs=4
  Merge2 : Merge
  Merge3 : Merge  Inputs=3
  Rigid Axle : Subsystem  TreatAsAtomicUnit=on
  Steering TV with TC : Subsystem  TreatAsAtomicUnit=on
  "Steering Wheel Saturation (per site) [deg] " : Constant  Value=10
  Terminator{,1..9} (10 alike) : Terminator
  VDC Complete : Subsystem  TreatAsAtomicUnit=on
  VDC without Longitudinal : Subsystem  TreatAsAtomicUnit=on
  Tq_RR [Nm] (0,inf) : Outport  VectorParamsAs1DForOutWhenUnconnected=off
  Tq_RL [Nm] (0,inf) : Outport  Port=2  VectorParamsAs1DForOutWhenUnconnected=off
  Tq_RRwc [Nm] (0,inf) : Outport  Port=3  VectorParamsAs1DForOutWhenUnconnected=off
  Tq_RLwc [Nm] (0,inf) : Outport  Port=4  VectorParamsAs1DForOutWhenUnconnected=off
  MaxTq_RR [Nm] (0,inf) : Outport  Port=5  VectorParamsAs1DForOutWhenUnconnected=off
  MaxTq_RL [Nm] (0,inf) : Outport  Port=6  VectorParamsAs1DForOutWhenUnconnected=off
  MaxFx_RR [N] (0,inf) : Outport  Port=7  VectorParamsAs1DForOutWhenUnconnected=off
  MaxFx_RL [N] (0,inf) : Outport  Port=8  VectorParamsAs1DForOutWhenUnconnected=off
  Throttle [0-1] (0-100%) : Outport  Port=9  VectorParamsAs1DForOutWhenUnconnected=off
  Fy_R [N] (0,inf) : Outport  Port=10  VectorParamsAs1DForOutWhenUnconnected=off
  Mass [kg] (0,inf) : Outport  Port=11  VectorParamsAs1DForOutWhenUnconnected=off
  Handling [-] (-inf,inf) : Outport  Port=12  VectorParamsAs1DForOutWhenUnconnected=off
  Flags [num5] : Outport  Port=13  VectorParamsAs1DForOutWhenUnconnected=off
  SKF_act : Outport  Port=14  VectorParamsAs1DForOutWhenUnconnected=off
  CKF_act : Outport  Port=15  VectorParamsAs1DForOutWhenUnconnected=off
  wires:
  VDC Complete/4(Tq_RLwc [Nm] (0,inf)) -> Tq_RLwc [Nm] (0,inf)/1
  VDC Complete/3(Tq_RRwc [Nm] (0,inf)) -> Tq_RRwc [Nm] (0,inf)/1
  VDC Complete/5(MaxTq_RR [Nm] (0,inf)) -> MaxTq_RR [Nm] (0,inf)/1
  VDC Complete/6(MaxTq_RL [Nm] (0,inf)) -> MaxTq_RL [Nm] (0,inf)/1
  VDC Complete/7(MaxFx_RR [N] (0,inf)) -> MaxFx_RR [N] (0,inf)/1
  VDC Complete/8(MaxFx_RL [N] (0,inf)) -> MaxFx_RL [N] (0,inf)/1
  VDC Complete/9(Throttle [0-1] (0-100%)) -> Throttle [0-1] (0-100%)/1
  VDC Complete/10(Fy_R [N] (0,inf)) -> Fy_R [N] (0,inf)/1
  VDC Complete/11(Mass [kg] (0,inf)) -> Mass [kg] (0,inf)/1
  VDC Complete/12(Handling [-] (-inf,inf)) -> Handling [-] (-inf,inf)/1
  VDC without Longitudinal/3(MaxTq_RR [Nm] (0,inf)) -> Terminator/1
  VDC without Longitudinal/4(MaxTq_RL [Nm] (0,inf)) -> Terminator1/1
  VDC without Longitudinal/5(MaxFx_RR [N] (0,inf)) -> Terminator2/1
  VDC without Longitudinal/6(MaxFx_RL [N] (0,inf)) -> Terminator3/1
  VDC without Longitudinal/7(Fy_R [N] (0,inf)) -> Terminator4/1
  VDC without Longitudinal/8(Throttle [0-1] (0-100%)) -> Terminator5/1
  VDC without Longitudinal/9(Mass [kg] (0,inf)) -> Terminator6/1
  VDC without Longitudinal/10(Handling [-] (-inf,inf)) -> Terminator7/1
  VDC without Longitudinal/11(Tq_RRwc [Nm] (0,inf)) -> Terminator8/1
  VDC without Longitudinal/12(Tq_RLwc [Nm] (0,inf)) -> Terminator9/1
  VDC Complete/13(Flags_[num5]) -> Flags [num5]/1
  Merge2/1 -> SKF_act/1
  Merge3/1 -> CKF_act/1
  "Steering Wheel Saturation (per site) [deg] "/1 -> Steering TV with TC/5("Steering Wheel Saturation (per site) "), VDC without Longitudinal/5(Steering Saturation (per site) [deg]), VDC Complete/5(Steering Saturation (per site) [deg])
  SKF_Initial/1 -> VDC without Longitudinal/6(SKF_initial), VDC Complete/6(SKF_Initial), Steering TV with TC/6(SKF_Initial)
  CKF_Initial/1 -> VDC Complete/7(CKF_Initial), VDC without Longitudinal/7(CKF_Initial), Steering TV with TC/7(CKF_Initial)
  Cte_SKF/1 -> VDC Complete/8(Cte_SKF), VDC without Longitudinal/8(Cte_SKF), Steering TV with TC/8(Cte_SKF)
  Cte_CKF/1 -> VDC Complete/9(Cte_CKF), VDC without Longitudinal/9(Cte_CKF), Steering TV with TC/9(Cte_CKF)
  Velocity_eRL [rad/s]/1 -> Steering TV with TC/10(Vel_eRL), VDC Complete/10(Velocity_eRL [rad/s]), VDC without Longitudinal/10(Velocity_eRL [rad/s])
  Velocity_eRR [rad/s]/1 -> Steering TV with TC/11(Vel_eRR), VDC Complete/11(Velocity_eRR [rad/s]), VDC without Longitudinal/11(Velocity_eRR [rad/s])
  Steering TV with TC/3(SKF_act) -> [SKF_act2]
  Steering TV with TC/4(CKF_act) -> [CKF_act2]
  VDC without Longitudinal/13(CKF_act) -> [CKF_act1]
  VDC Complete/14(SKF_act) -> [SKF_act0]
  VDC Complete/15(CKF_act) -> [CKF_act0]
  [CKF_act1] -> Merge3/2
  [CKF_act0] -> Merge3/1
  [CKF_act2] -> Merge3/3
  [SKF_act0] -> Merge2/1
  [SKF_act2] -> Merge2/2
  FAILURE MODE/1 -> VDC Complete/Action
  FAILURE MODE/2 -> VDC without Longitudinal/Action
  FAILURE MODE/3 -> Steering TV with TC/Action
  FAILURE MODE/4 -> Rigid Axle/Action
  Brake Pedal (0-1) [-]/1 -> VDC Complete/19(Brake Pedal (0-1) [-]), VDC without Longitudinal/19(Brake Pedal (0-1) [-]), [Bp]
  FR_Susp [N]/1 -> VDC Complete/13(FR_Susp [N]), VDC without Longitudinal/13(FR_Susp [N])
  FL_Susp [N]/1 -> VDC Complete/14(FL_Susp [N]), VDC without Longitudinal/14(FL_Susp [N])
  RR_Susp [N]/1 -> VDC Complete/15(RR_Susp [N]), VDC without Longitudinal/15(RR_Susp [N])
  RL_Susp [N]/1 -> VDC Complete/16(RL_Susp [N]), VDC without Longitudinal/16(RL_Susp [N])
  Regenerative Enable [0,1]/1 -> [Regen_enable], VDC Complete/17(Regenerative Enable [0,1]), VDC without Longitudinal/17(Regenerative Enable [0,1])
  Max Regen Torque [Nm]/1 -> [Max_Regen_Tq], VDC Complete/18(Max Regen Torque [Nm]), VDC without Longitudinal/18(Max Regen Torque [Nm])
  Steering TV with TC/1(Tq_RR_E2 [Nm] (0,inf)) -> [Tq_RR_E2]
  Steering TV with TC/2(Tq_RL_E2 [Nm] (0,inf)) -> [Tq_RL_E2]
  VDC without Longitudinal/1(Tq_RR_E1 [Nm] (0,inf)) -> [Tq_RR_E1]
  VDC Complete/1(Tq_RR_E0 [Nm] (0,inf)) -> [Tq_RR_E0]
  VDC Complete/2(Tq_RL_E0 [Nm] (0,inf)) -> [Tq_RL_E0]
  Merge Tq_RR/1 -> Display/1, Tq_RR [Nm] (0,inf)/1
  Rigid Axle/1(Tq_RR_E3 [Nm] (0,inf)) -> [Tq_RR_E3]
  Rigid Axle/2(Tq_RL_E3 [Nm] (0,inf)) -> [Tq_RL_E3]
  Merge Tq_RL/1 -> Display1/1, Tq_RL [Nm] (0,inf)/1
  [Tq_RR_E0] -> Merge Tq_RR/4
  [Tq_RR_E1] -> Merge Tq_RR/3
  [Tq_RR_E2] -> Merge Tq_RR/2
  [Tq_RR_E3] -> Merge Tq_RR/1
  [Tq_RL_E0] -> Merge Tq_RL/4
  [Tq_RL_E1] -> Merge Tq_RL/3
  [Tq_RL_E2] -> Merge Tq_RL/2
  [Tq_RL_E3] -> Merge Tq_RL/1
  [Bp] -> Steering TV with TC/12(Bp)
  [Max_Regen_Tq] -> Steering TV with TC/13(Max_Regen_Tq)
  [Regen_enable] -> Steering TV with TC/14(Regen_enable)
  If/1 -> Automatic Failure Mode/Action
  FAILURE_MODE1/1 -> Automatic Failure Mode/1(In1)
  If/2 -> Manual Failure Mode Selection/Action
  Constant/1 -> [FM_select], If/1
  [FM_select] -> Manual Failure Mode Selection/1(In1)
  Merge/1 -> FAILURE MODE/1
  Automatic Failure Mode/1(Out1) -> Merge/1
  Manual Failure Mode Selection/1(Out1) -> Merge/2
  VDC without Longitudinal/2(Tq_RL_E1 [Nm] (0,inf)) -> [Tq_RL_E1]
  Ellipse_acc(ax,ay,az)/1 -> [ellipse_acc_ax_ay_az]
  Ellipse_vel(vx,vy,vz)/1 -> [ellipse_vel_vx_vy_vz]
  Ellipse_gyro(gx,gy,gz)/1 -> [ellipse_gyro_gx_gy_gz]
  Ellipse_yaw/1 -> [ellipse_yaw]
  Ellipse_pitch/1 -> [ellipse_pitch]
  Ellipse_roll/1 -> [ellipse_roll]
  [ellipse_acc_ax_ay_az] -> VDC without Longitudinal/12(Ellipse_acc_ax_ay_az)
  [ellipse_acc_ax_ay_az] -> VDC Complete/12(Ellipse_acc)
  [ellipse_gyro_gx_gy_gz] -> VDC Complete/20(Gyro_Ellipse)
  [ellipse_vel_vx_vy_vz] -> VDC Complete/21(Ellipse_vel)
  Gas Pedal (0-1) [-]/1 -> [gas_pedal_0_1]
  [gas_pedal_0_1] -> Rigid Axle/3(Gas Pedal [0-1])
  [gas_pedal_0_1] -> Steering TV with TC/3(Gas Pedal [0-1])
  [gas_pedal_0_1] -> VDC without Longitudinal/3(Gas Pedal (0-1) [-])
  [gas_pedal_0_1] -> VDC Complete/3(Gas Pedal (0-1) [-])
  Ap_Sat_Up/1 -> [ap_sat_up]
  Ap_Sat_Down/1 -> [ap_sat_down]
  [ap_sat_up] -> Rigid Axle/1("Ap_Sat_up ")
  [ap_sat_down] -> Rigid Axle/2(Ap_Sat_down)
  [ap_sat_up] -> Steering TV with TC/1("Ap_Sat_up ")
  [ap_sat_down] -> Steering TV with TC/2(Ap_Sat_down)
  [ap_sat_up] -> VDC without Longitudinal/1(Ap_Sat_Up [-])
  [ap_sat_down] -> VDC without Longitudinal/2(Ap_Sat_Down [-])
  [ap_sat_down] -> VDC Complete/2(Ap_Sat_Down [-])
  [ap_sat_up] -> VDC Complete/1(Ap_Sat_Up [-])
  Steering_Angle [deg]/1 -> Gain/1
  Gain/1 -> [steering_angle_normalized]
  [steering_angle_normalized] -> Steering TV with TC/4(Steering_Angle [deg])
  [steering_angle_normalized] -> VDC without Longitudinal/4(Steering_Angle [deg])
  [steering_angle_normalized] -> VDC Complete/4(Steering_Angle [deg])
